simulink model "Model_5ms"  (Simulink 7.7)
settings: Solver=ode45  StartTime=0.0  StopTime=10.0  RelTol=1e-3
undefined symbols (not defined in the file): DiscIntNeverNeededParam
libraries: simulink x3, simulink_extras x2
settings Model: Creator=carsim  LastModifiedBy=jporter
settings DebuggingCC: FcnCallInpInsideContextMsg=Enable All

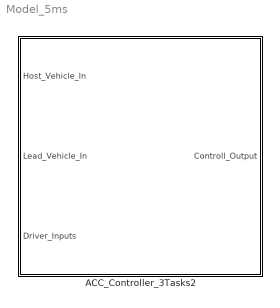
== system Model_5ms ==
  ACC_Controller_3Tasks2 : Subsystem

== system Model_5ms/ACC_Controller_3Tasks2 ==
  Host_Vehicle_In : Inport
  Lead_Vehicle_In : Inport  Port=2
  Driver_Inputs : Inport  Port=3
  HighLevelController : Subsystem
  Instrument Cluster : Subsystem
  LowLevel : Subsystem
  Mux2 : Mux  Inputs=5
  Controll_Output : Outport
  wires:
  Instrument Cluster/1(Detect) -> Mux2/3
  Instrument Cluster/2(Distance_actual) -> Mux2/4
  Mux2/1 -> Controll_Output/1
  Host_Vehicle_In/1 -> Instrument Cluster/1(Host_Vehicle_In)
  Driver_Inputs/1 -> Instrument Cluster/3(Driver_Inputs)
  Lead_Vehicle_In/1 -> Instrument Cluster/2(Lead_Vehicle_In)
  HighLevelController/1(To_LowLevelController) -> LowLevel/1(Lowlevel_inputs_from_HighLevel)
  Instrument Cluster/3(To_High_Level_Controller) -> HighLevelController/1(High_Level_inputs)
  LowLevel/1(Throttle_Angle) -> Instrument Cluster/4(Throttle_ang_in)
  LowLevel/2(P_mc_Brake) -> Instrument Cluster/5(P_mc_brake_in)
  LowLevel/3(desired_Range) -> Instrument Cluster/6(des_range_in)
  Instrument Cluster/4(Throttle_ang_out) -> Mux2/1
  Instrument Cluster/5(P_mc_brake_out) -> Mux2/2
  Instrument Cluster/6(des_range_out) -> Mux2/5

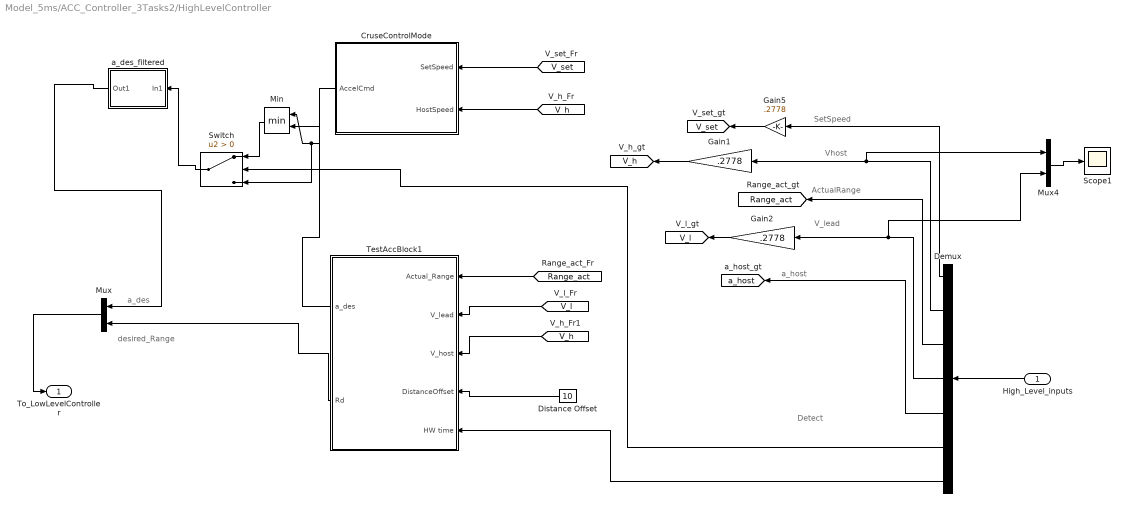
== system Model_5ms/ACC_Controller_3Tasks2/HighLevelController ==
  note: SetSpeed
  note: Vhost
  note: ActualRange
  note: V_lead
  note: a_host
  note: Detect
  note: a_des
  note: desired_Range
  High_Level_inputs : Inport
  CruseControlMode : Subsystem
  Demux : Demux  Outputs=7
  Distance Offset : Constant  Value=10
  Gain1 : Gain  Gain=.2778
  Gain2 : Gain  Gain=.2778
  Gain5 : Gain  Gain=.2778
  Min : MinMax  Inputs=2
  Mux : Mux  Inputs=2
  Mux4 : Mux  Inputs=2
  Scope1 : Scope
      settings: YMin=60  YMax=60.3
  Switch : Switch  Criteria=u2 > Threshold
  TestAccBlock1 : Subsystem
  a_des_filtered : Subsystem
  To_LowLevelController : Outport
  tag scope: Range_act=global, V_h=global, V_l=global, V_set=global, a_host=global
  wires:
  [V_h] -> TestAccBlock1/3(V_host)
  [V_h] -> CruseControlMode/2(HostSpeed)
  [V_set] -> CruseControlMode/1(SetSpeed)
  [Range_act] -> TestAccBlock1/1(Actual_Range)
  [V_l] -> TestAccBlock1/2(V_lead)
  Distance Offset/1 -> TestAccBlock1/4(DistanceOffset)
  CruseControlMode/1(AccelCmd) -> Switch/3, Min/1
  a_des_filtered/1(Out1) -> Mux/1
  TestAccBlock1/2(Rd) -> Mux/2
  TestAccBlock1/1(a_des) -> Min/2
  Switch/1 -> a_des_filtered/1(In1)
  Min/1 -> Switch/1
  Gain5/1 -> [V_set]
  Gain1/1 -> [V_h]
  Gain2/1 -> [V_l]
  Demux/7 -> TestAccBlock1/5(HW time)
  Demux/1 -> Gain5/1
  Demux/2 -> Gain1/1, Mux4/1
  Demux/3 -> [Range_act]
  Demux/4 -> Gain2/1, Mux4/2
  Demux/5 -> [a_host]
  Demux/6 -> Switch/2
  Mux/1 -> To_LowLevelController/1
  High_Level_inputs/1 -> Demux/1
  Mux4/1 -> Scope1/1

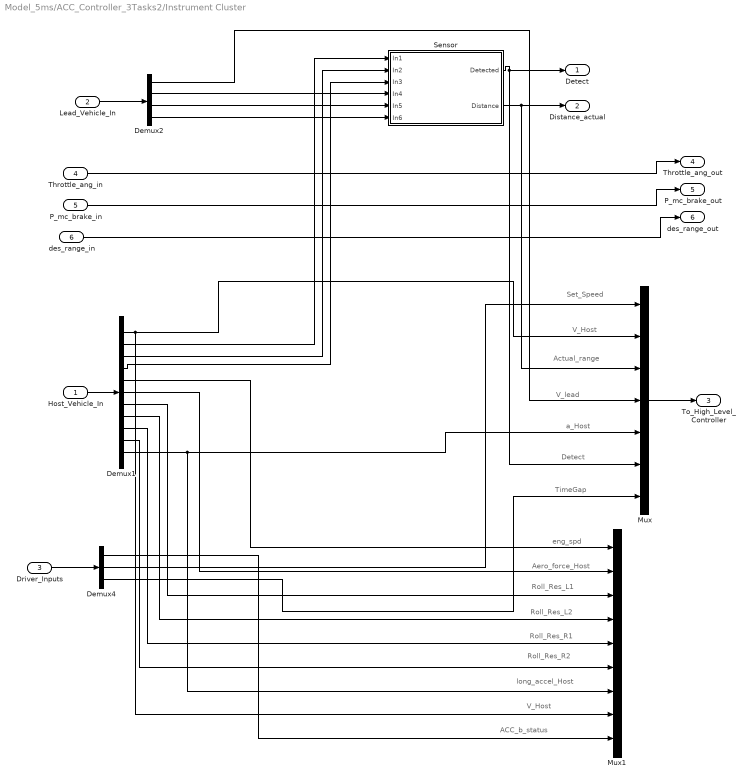
== system Model_5ms/ACC_Controller_3Tasks2/Instrument Cluster ==
  note: Set_Speed
  note: V_Host
  note: Actual_range
  note: V_lead
  note: a_Host
  note: Detect
  note: TimeGap
  note: eng_spd
  note: Aero_force_Host
  note: Roll_Res_L1
  note: Roll_Res_L2
  note: Roll_Res_R1
  note: Roll_Res_R2
  note: long_accel_Host
  note: V_Host
  note: ACC_b_status
  Host_Vehicle_In : Inport
  Lead_Vehicle_In : Inport  Port=2
  Driver_Inputs : Inport  Port=3
  Throttle_ang_in : Inport  Port=4
  P_mc_brake_in : Inport  Port=5
  des_range_in : Inport  Port=6
  Demux1 : Demux  Outputs=11
  Demux2 : Demux
  Demux4 : Demux  Outputs=3
  Mux : Mux  Inputs=7
  Mux1 : Mux  Inputs=9
  Sensor : Subsystem  mask{S_ANGLE=30, S_DISTANCE=100}
      mask prompts: S_ANGLE "View Angle (deg)"; S_DISTANCE "Distance Range (m)"
      mask help:
      | An example of a radar sensor. It can detect the distance between the sensor and another object according its position (Xo, Yo).
      |
      | Input parameters are View Angle(deg) and radar detectable distance(m).
      mask init:
      | d_ang= str2double(S_ANGLE)/2;
      | set_param([gcb '/View Angle'], 'Threshold', sprintf('%0.2f', d_ang));
      | set_param([gcb '/L-Radar'], 'Value', S_DISTANCE);
  Detect : Outport
  Distance_actual : Outport  Port=2
  To_High_Level_Controller : Outport  Port=3
  Throttle_ang_out : Outport  Port=4
  P_mc_brake_out : Outport  Port=5
  des_range_out : Outport  Port=6
  wires:
  Sensor/2(Distance) -> Distance_actual/1, Mux/3
  Sensor/1(Detected) -> Detect/1, Mux/6
  Demux4/1 -> Mux1/9
  Demux4/2 -> Mux/1
  Demux4/3 -> Mux/7
  Driver_Inputs/1 -> Demux4/1
  Demux1/1 -> Mux1/8, Mux/2
  Demux1/2 -> Sensor/1(In1)
  Demux1/3 -> Sensor/2(In2)
  Demux1/4 -> Sensor/3(In3)
  Demux1/5 -> Mux1/1
  Demux1/6 -> Mux1/2
  Demux1/7 -> Mux1/3
  Demux1/8 -> Mux1/4
  Demux1/9 -> Mux1/5
  Demux1/10 -> Mux1/6
  Demux1/11 -> Mux/5, Mux1/7
  Host_Vehicle_In/1 -> Demux1/1
  Lead_Vehicle_In/1 -> Demux2/1
  Demux2/2 -> Sensor/4(In4)
  Demux2/3 -> Sensor/5(In5)
  Demux2/4 -> Sensor/6(In6)
  Demux2/1 -> Mux/4
  Mux/1 -> To_High_Level_Controller/1
  Throttle_ang_in/1 -> Throttle_ang_out/1
  P_mc_brake_in/1 -> P_mc_brake_out/1
  des_range_in/1 -> des_range_out/1

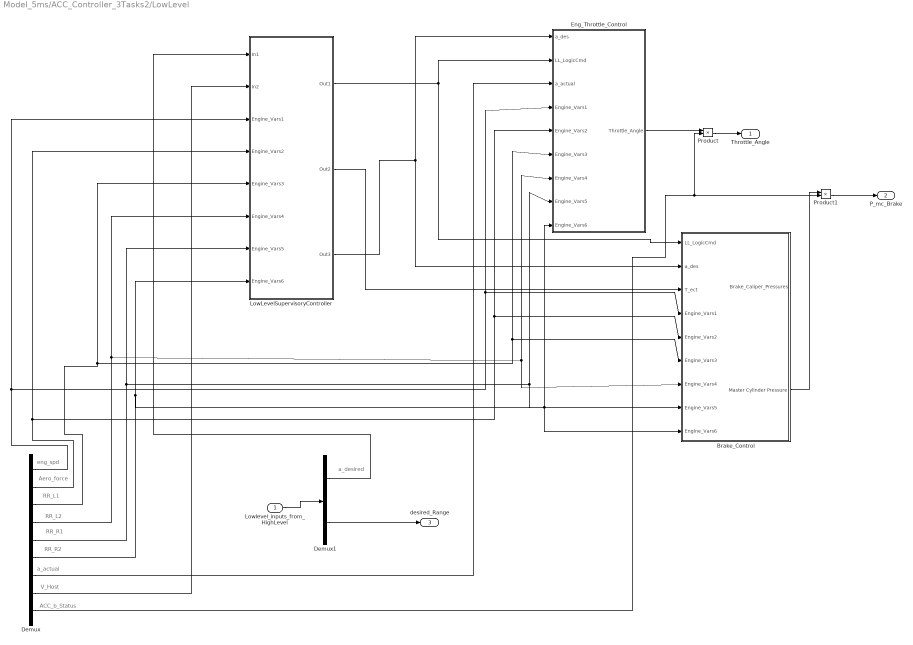
== system Model_5ms/ACC_Controller_3Tasks2/LowLevel ==
  note: eng_spd
  note: Aero_force
  note: RR_L1
  note: RR_L2
  note: RR_R1
  note: RR_R2
  note: a_desired
  note: a_actual
  note: V_Host
  note: ACC_b_Status
  Lowlevel_inputs_from_HighLevel : Inport
  Brake_Control : Subsystem
  Demux : Demux  Outputs=9
  Demux1 : Demux  Outputs=2
  Eng_Throttle_Control : Subsystem
  LowLevelSupervisoryController : Subsystem
  Product : Product  RndMeth=Zero
  Product1 : Product  RndMeth=Zero
  Throttle_Angle : Outport
  P_mc_Brake : Outport  Port=2
  desired_Range : Outport  Port=3
  wires:
  Demux/3 -> Eng_Throttle_Control/6(Engine_Vars3), Brake_Control/6(Engine_Vars3), LowLevelSupervisoryController/5(Engine_Vars3)
  Demux/5 -> Eng_Throttle_Control/8(Engine_Vars5), Brake_Control/8(Engine_Vars5), LowLevelSupervisoryController/7(Engine_Vars5)
  LowLevelSupervisoryController/1(Out1) -> Brake_Control/1(LL_LogicCmd), Eng_Throttle_Control/2(LL_LogicCmd)
  LowLevelSupervisoryController/3(Out3) -> Brake_Control/2(a_des), Eng_Throttle_Control/1(a_des)
  LowLevelSupervisoryController/2(Out2) -> Brake_Control/3(T_ect)
  Product/1 -> Throttle_Angle/1
  Product1/1 -> P_mc_Brake/1
  Eng_Throttle_Control/1(Throttle_Angle) -> Product/1
  Brake_Control/2(Master Cylinder Pressure) -> Product1/1
  Demux/1 -> Brake_Control/4(Engine_Vars1), Eng_Throttle_Control/4(Engine_Vars1), LowLevelSupervisoryController/3(Engine_Vars1)
  Demux/2 -> Eng_Throttle_Control/5(Engine_Vars2), Brake_Control/5(Engine_Vars2), LowLevelSupervisoryController/4(Engine_Vars2)
  Demux/4 -> Eng_Throttle_Control/7(Engine_Vars4), Brake_Control/7(Engine_Vars4), LowLevelSupervisoryController/6(Engine_Vars4)
  Demux/6 -> Eng_Throttle_Control/9(Engine_Vars6), Brake_Control/9(Engine_Vars6), LowLevelSupervisoryController/8(Engine_Vars6)
  Demux/9 -> Product/2, Product1/2
  Demux1/2 -> desired_Range/1
  Demux1/1 -> LowLevelSupervisoryController/1(In1)
  Demux/7 -> Eng_Throttle_Control/3(a_actual)
  Demux/8 -> LowLevelSupervisoryController/2(In2)
  Lowlevel_inputs_from_HighLevel/1 -> Demux1/1

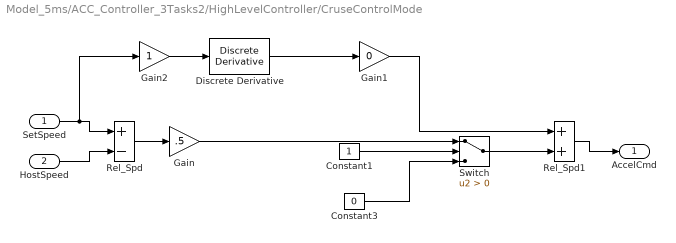
== system Model_5ms/ACC_Controller_3Tasks2/HighLevelController/CruseControlMode ==
  SetSpeed : Inport
  HostSpeed : Inport  Port=2
  Constant1 : Constant
  Constant3 : Constant  Value=0
  Discrete Derivative : simulink/Discrete/Discrete Derivative  gainval=.1  ICPrevScaledInput=0.0  InputProcessing=Inherited  OutMin=[]  OutMax=[]  OutDataType=fixdt(1, 16)  OutScaling=2^-10  DoSatur=off
  Gain : Gain  Gain=.5
  Gain1 : Gain  Gain=0
  Gain2 : Gain  SampleTime=.005
  Rel_Spd : Sum  Inputs=+-
  Rel_Spd1 : Sum
  Switch : Switch  Criteria=u2 > Threshold
  AccelCmd : Outport
  wires:
  SetSpeed/1 -> Rel_Spd/1, Gain2/1
  HostSpeed/1 -> Rel_Spd/2
  Rel_Spd/1 -> Gain/1
  Gain/1 -> Switch/1
  Constant3/1 -> Switch/3
  Switch/1 -> Rel_Spd1/2
  Constant1/1 -> Switch/2
  Gain1/1 -> Rel_Spd1/1
  Discrete Derivative/1 -> Gain1/1
  Rel_Spd1/1 -> AccelCmd/1
  Gain2/1 -> Discrete Derivative/1

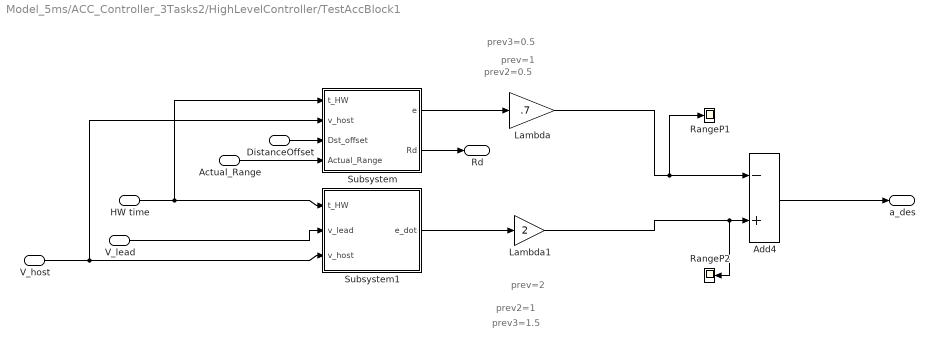
== system Model_5ms/ACC_Controller_3Tasks2/HighLevelController/TestAccBlock1 ==
  note: prev=1
  note: prev=2
  note: prev2=0.5
  note: prev2=1
  note: prev3=1.5
  note: prev3=0.5
  Actual_Range : Inport
  V_lead : Inport  Port=2
  V_host : Inport  Port=3
  DistanceOffset : Inport  Port=4
  HW time : Inport  Port=5
  Add4 : Sum  Inputs=-+
  Lambda : Gain  Gain=.7
  Lambda1 : Gain  Gain=2
  RangeP1 : Scope
      settings: TickLabels=on  TimeRange=50  YMin=-2  YMax=3.75  SaveName=ScopeData32  DataFormat=Array  SampleTime=100
  RangeP2 : Scope
      settings: TickLabels=on  TimeRange=50  YMin=-2  YMax=3.75  SaveName=ScopeData33  DataFormat=Array  SampleTime=100
  Subsystem : Subsystem
  Subsystem1 : Subsystem
  a_des : Outport
  Rd : Outport  Port=2
  wires:
  V_host/1 -> Subsystem1/3(v_host), Subsystem/2(v_host)
  HW time/1 -> Subsystem1/1(t_HW), Subsystem/1(t_HW)
  V_lead/1 -> Subsystem1/2(v_lead)
  Subsystem1/1(e_dot) -> Lambda1/1
  Lambda/1 -> Add4/1, RangeP1/1
  Add4/1 -> a_des/1
  Subsystem/1(e) -> Lambda/1
  Actual_Range/1 -> Subsystem/4(Actual_Range)
  DistanceOffset/1 -> Subsystem/3(Dst_offset)
  Subsystem/2(Rd) -> Rd/1
  Lambda1/1 -> Add4/2, RangeP2/1

== system Model_5ms/ACC_Controller_3Tasks2/HighLevelController/a_des_filtered ==
  In1 : Inport
  Discrete Transfer Fcn : DiscreteTransferFcn  Numerator=[0,0.00120910427425029,0.00116946476028127]  Denominator=[1,-1.90245884900143,0.904837418035960]  SampleTime=.005
  Saturation : Saturate  UpperLimit=2  LowerLimit=-3
  Out1 : Outport
  wires:
  In1/1 -> Saturation/1
  Discrete Transfer Fcn/1 -> Out1/1
  Saturation/1 -> Discrete Transfer Fcn/1

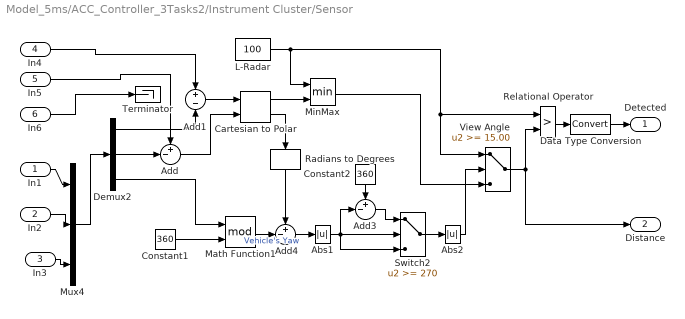
== system Model_5ms/ACC_Controller_3Tasks2/Instrument Cluster/Sensor ==
  In1 : Inport
  In2 : Inport  Port=2
  In3 : Inport  Port=3
  In4 : Inport  Port=4
  In5 : Inport  Port=5
  In6 : Inport  Port=6
  Abs1 : Abs
  Abs2 : Abs
  Add : Sum  Inputs=+-|
  Add1 : Sum  Inputs=+-
  Add3 : Sum  Inputs=+-|
  Add4 : Sum  Inputs=+-|
  Cartesian to Polar : simulink_extras/Transformations/Cartesian to Polar
  Constant1 : Constant  Value=360
  Constant2 : Constant  Value=360
  Data Type Conversion : DataTypeConversion  RndMeth=Zero
  Demux2 : Demux  Outputs=3
  L-Radar : Constant  Value=100
  Math Function1 : Math  Operator=mod  SaturateOnIntegerOverflow=on
  MinMax : MinMax  Inputs=2  SaturateOnIntegerOverflow=on  InputSameDT=on
  Mux4 : Mux  Inputs=3
  Radians to Degrees : simulink_extras/Transformations/Radians to Degrees
  Relational Operator : RelationalOperator  Operator=>  OutDataTypeStr=boolean
  Switch2 : Switch  Threshold=270
  Terminator : Terminator
  View Angle : Switch  Threshold=15.00
  Detected : Outport
  Distance : Outport  Port=2
  wires:
  Demux2/3 -> Math Function1/1
  Constant1/1 -> Math Function1/2
  Add/1 -> Cartesian to Polar/2
  Add1/1 -> Cartesian to Polar/1
  Demux2/1 -> Add1/2
  In4/1 -> Add1/1
  Demux2/2 -> Add/2
  In5/1 -> Add/1
  In6/1 -> Terminator/1
  Math Function1/1 -> Add4/2  "Vehicle's Yaw"
  Add4/1 -> Abs1/1
  Abs1/1 -> Switch2/2, Add3/2, Switch2/3
  Add3/1 -> Switch2/1
  Constant2/1 -> Add3/1
  L-Radar/1 -> MinMax/1, View Angle/1, Relational Operator/1
  MinMax/1 -> View Angle/3
  Switch2/1 -> Abs2/1
  Abs2/1 -> View Angle/2
  View Angle/1 -> Distance/1, Relational Operator/2
  Relational Operator/1 -> Data Type Conversion/1
  Data Type Conversion/1 -> Detected/1
  Radians to Degrees/1 -> Add4/1
  Cartesian to Polar/1 -> MinMax/2
  Cartesian to Polar/2 -> Radians to Degrees/1
  Mux4/1 -> Demux2/1
  In1/1 -> Mux4/1
  In2/1 -> Mux4/2
  In3/1 -> Mux4/3

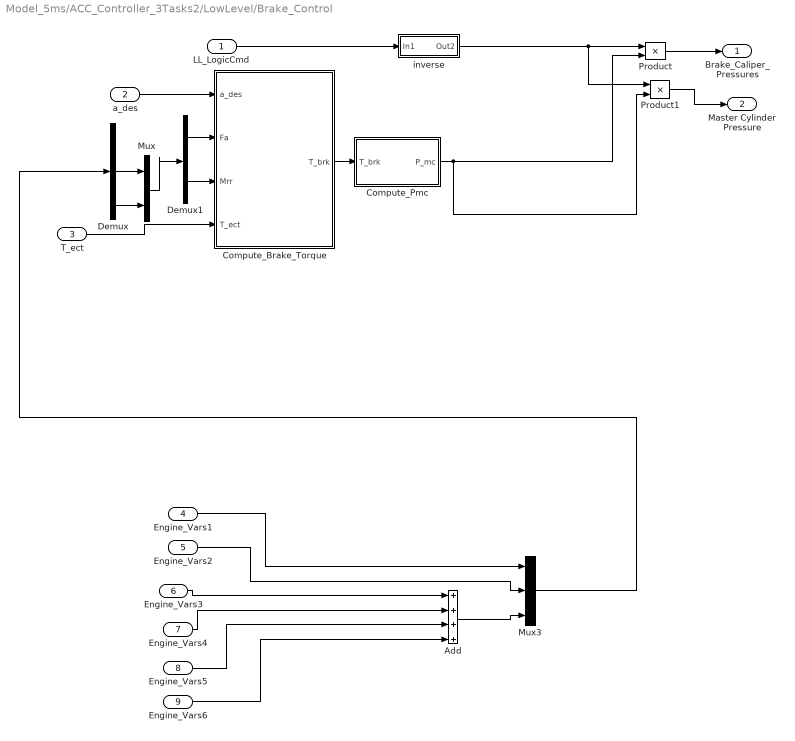
== system Model_5ms/ACC_Controller_3Tasks2/LowLevel/Brake_Control ==
  LL_LogicCmd : Inport
  a_des : Inport  Port=2
  T_ect : Inport  Port=3
  Engine_Vars1 : Inport  Port=4
  Engine_Vars2 : Inport  Port=5
  Engine_Vars3 : Inport  Port=6
  Engine_Vars4 : Inport  Port=7
  Engine_Vars5 : Inport  Port=8
  Engine_Vars6 : Inport  Port=9
  Add : Sum  Inputs=++++
  Compute_Brake_Torque : Stateflow chart  TreatAsAtomicUnit=on
  Compute_Pmc : Stateflow chart  TreatAsAtomicUnit=on
  Demux : Demux  Outputs=3
  Demux1 : Demux  Outputs=2
  Mux : Mux  Inputs=2
  Mux3 : Mux  Inputs=3
  Product : Product  RndMeth=Zero
  Product1 : Product  RndMeth=Zero
  inverse : Subsystem
  Brake_Caliper_Pressures : Outport
  Master Cylinder Pressure : Outport  Port=2
  wires:
  LL_LogicCmd/1 -> inverse/1(In1)
  inverse/1(Out2) -> Product/1, Product1/1
  Product/1 -> Brake_Caliper_Pressures/1
  Mux3/1 -> Demux/1
  Compute_Pmc/1(P_mc) -> Product1/2, Product/2
  Product1/1 -> Master Cylinder Pressure/1
  Compute_Brake_Torque/1(T_brk) -> Compute_Pmc/1(T_brk)
  Demux1/1 -> Compute_Brake_Torque/2(Fa)
  Demux1/2 -> Compute_Brake_Torque/3(Mrr)
  Demux/3 -> Mux/2
  Demux/2 -> Mux/1
  Mux/1 -> Demux1/1
  T_ect/1 -> Compute_Brake_Torque/4(T_ect)
  a_des/1 -> Compute_Brake_Torque/1(a_des)
  Engine_Vars2/1 -> Mux3/2
  Engine_Vars3/1 -> Add/1
  Engine_Vars4/1 -> Add/2
  Add/1 -> Mux3/3
  Engine_Vars1/1 -> Mux3/1
  Engine_Vars5/1 -> Add/3
  Engine_Vars6/1 -> Add/4

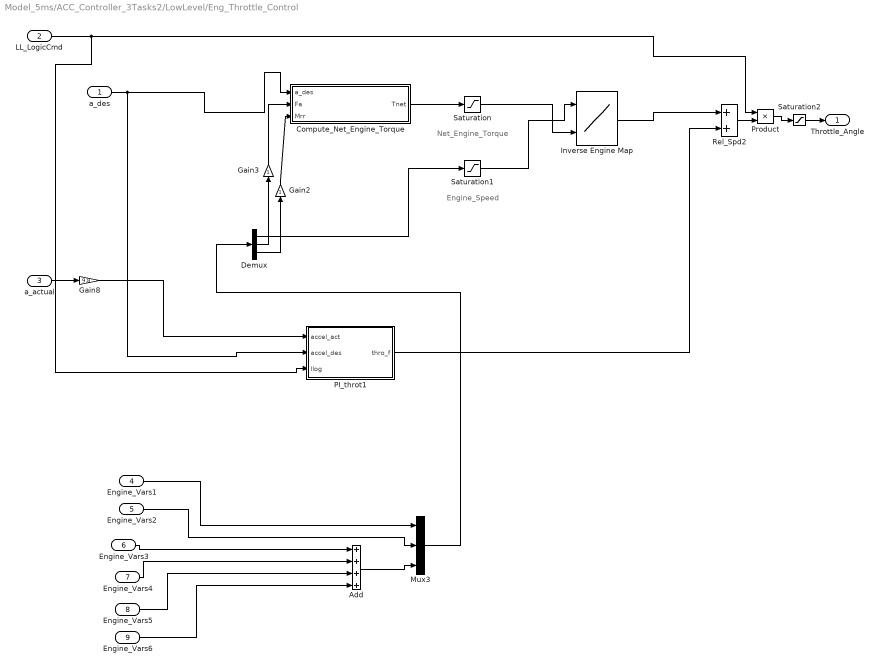
== system Model_5ms/ACC_Controller_3Tasks2/LowLevel/Eng_Throttle_Control ==
  note: Net_Engine_Torque
  note: Engine_Speed
  a_des : Inport
  LL_LogicCmd : Inport  Port=2
  a_actual : Inport  Port=3
  Engine_Vars1 : Inport  Port=4
  Engine_Vars2 : Inport  Port=5
  Engine_Vars3 : Inport  Port=6
  Engine_Vars4 : Inport  Port=7
  Engine_Vars5 : Inport  Port=8
  Engine_Vars6 : Inport  Port=9
  Add : Sum  Inputs=++++
  Compute_Net_Engine_Torque : Stateflow chart  TreatAsAtomicUnit=on
  Demux : Demux  Outputs=3
  Gain2 : Gain
  Gain3 : Gain
  Gain8 : Gain  Gain=9.8
  Inverse Engine Map : Lookup_n-D  BreakpointsForDimension1=|  BreakpointsForDimension2=[-131:12:514]  Table=[0,0,0,0,0,0,0,0,0,0,0,0,0,0,0,0.0100000000000000,0.0200000000000000,0.0400000000000000,0.0500000000000000,0.0700000000000000,0.0800000000000000,0.0900000000000000,0.110000000000000,0.120000000000000,0.140000000000000,0.160000000000000,0.950000000000000,0.950000000000000,0.950000000000000,0.950000000000000,0.950000000000000,0.950000000000000,0.950000000000000,0.950000000000000,0.950000000000000,0.950000000000000,0.950000000000000,0.950000000000000,0.950000000000000,0.950000000000000,0.950000000000000,0.950000000000000,0.950000000000000,0.950000000000000,0.950000000000000,0.950000000000000,0.950000000000000,0.950000000000000,0.950000000000000,0.950000000000000,0.950000000000000,0.950000000000000,0.950000000000000,0.950000000000000;0,0,0,0,0,0,0,0,0,0,0,0,0,0,0,0,0.0100000000000000,0.0200000000000000,0.0300000000000000,0.0500000000000000,0.0600000000000000,0.0700000000000000,0.0800000000000000,0.0900000000000000,0.100000000000000,0.110000000000000,0.120000000000000,0.120000000000000,0.130000000000000,0.140000000000000,0.150000000000000,0.180000000000000,1,1,1,1,1,1,1,1,1,1,1,1,1,1,1,1,1,1,1,1,1,1;0,0,0,0,0,0,0,0,0,0,0,0,0.0100000000000000,0.0200000000000000,0.0300000000000000,0.0300000000000000,0.0400000000000000,0.0500000000000000,0.0600000000000000,0.0700000000000000,0.0800000000000000,0.0800000000000000,0.0900000000000000,0.100000000000000,0.110000000000000,0.110000000000000,0.120000000000000,0.120000000000000,0.130000000000000,0.140000000000000,0.140000000000000,0.150000000000000,0.170000000000000,0.190000000000000,0.690000000000000,0.850000000000000,0.850000000000000,0.850000000000000,0.850000000000000,0.850000000000000,0.850000000000000,0.850000000000000,0.850000000000000,0.850000000000000,0.850000000000000,0.850000000000000,0.850000000000000,0.850000000000000,0.850000000000000,0.850000000000000,0.850000000000000,0.850000000000000,0.850000000000000,0.850000000000000;0,0,0,0,0,0,0,0,0,0,0,0.0100000000000000,0.0200000000000000,0.0300000000000000,0.0400000000000000,0.0500000000000000,0.0600000000000000,0.0700000000000000,0.0800000000000000,0.0800000000000000,0.0900000000000000,0.100000000000000,0.100000000000000,0.110000000000000,0.110000000000000,0.120000000000000,0.120000000000000,0.120000000000000,0.130000000000000,0.130000000000000,0.130000000000000,0.140000000000000,0.140000000000000,0.140000000000000,0.150000000000000,0.150000000000000,0.170000000000000,0.180000000000000,0.190000000000000,0.260000000000000,0.410000000000000,0.850000000000000,0.850000000000000,0.850000000000000,0.850000000000000,0.850000000000000,0.850000000000000,0.850000000000000,0.850000000000000,0.850000000000000,0.850000000000000,0.850000000000000,0.850000000000000,0.850000000000000;0,0,0,0,0,0,0,0,0,0,0.0100000000000000,0.0200000000000000,0.0400000000000000,0.0500000000000000,0.0600000000000000,0.0700000000000000,0.0800000000000000,0.0900000000000000,0.100000000000000,0.100000000000000,0.110000000000000,0.110000000000000,0.110000000000000,0.120000000000000,0.120000000000000,0.120000000000000,0.130000000000000,0.130000000000000,0.130000000000000,0.130000000000000,0.140000000000000,0.140000000000000,0.140000000000000,0.150000000000000,0.150000000000000,0.160000000000000,0.170000000000000,0.180000000000000,0.180000000000000,0.190000000000000,0.220000000000000,0.310000000000000,0.430000000000000,0.960000000000000,1,1,1,1,1,1,1,1,1,1;0,0,0,0,0,0,0,0,0,0.0100000000000000,0.0200000000000000,0.0400000000000000,0.0600000000000000,0.0700000000000000,0.0900000000000000,0.100000000000000,0.100000000000000,0.110000000000000,0.110000000000000,0.110000000000000,0.120000000000000,0.120000000000000,0.120000000000000,0.130000000000000,0.130000000000000,0.130000000000000,0.130000000000000,0.140000000000000,0.140000000000000,0.140000000000000,0.150000000000000,0.150000000000000,0.150000000000000,0.160000000000000,0.160000000000000,0.170000000000000,0.180000000000000,0.180000000000000,0.190000000000000,0.190000000000000,0.200000000000000,0.240000000000000 ...(+10120 chars)]  RndMeth=Simplest  InputSameDT=on
      | [517
      | 633
      | 750
      | 1107
      | 1463
      | 1820
      | 2177
      | 2533
      | 2890
      | 3247
      | 3603
      | 3960
      | 4317
      | 4673
      | 5030
      | 5387
      | 5743
      | 6100]
  Mux3 : Mux  Inputs=3
  PI_throt1 : Subsystem
  Product : Product  RndMeth=Zero
  Rel_Spd2 : Sum
  Saturation : Saturate  UpperLimit=514  LowerLimit=-131
  Saturation1 : Saturate  UpperLimit=6100  LowerLimit=0
  Saturation2 : Saturate  UpperLimit=1  LowerLimit=0
  Throttle_Angle : Outport
  wires:
  LL_LogicCmd/1 -> PI_throt1/3(llog), Product/1
  Inverse Engine Map/1 -> Rel_Spd2/1
  Demux/1 -> Saturation1/1
  Compute_Net_Engine_Torque/1(Tnet) -> Saturation/1
  a_des/1 -> Compute_Net_Engine_Torque/1(a_des), PI_throt1/2(accel_des)
  Demux/2 -> Gain3/1
  Demux/3 -> Gain2/1
  Gain2/1 -> Compute_Net_Engine_Torque/3(Mrr)
  Gain3/1 -> Compute_Net_Engine_Torque/2(Fa)
  Saturation/1 -> Inverse Engine Map/2
  Saturation1/1 -> Inverse Engine Map/1
  PI_throt1/1(thro_f) -> Rel_Spd2/2
  Rel_Spd2/1 -> Product/2
  Saturation2/1 -> Throttle_Angle/1
  Product/1 -> Saturation2/1
  a_actual/1 -> Gain8/1
  Gain8/1 -> PI_throt1/1(accel_act)
  Engine_Vars2/1 -> Mux3/2
  Engine_Vars3/1 -> Add/1
  Engine_Vars4/1 -> Add/2
  Add/1 -> Mux3/3
  Engine_Vars1/1 -> Mux3/1
  Engine_Vars5/1 -> Add/3
  Engine_Vars6/1 -> Add/4
  Mux3/1 -> Demux/1

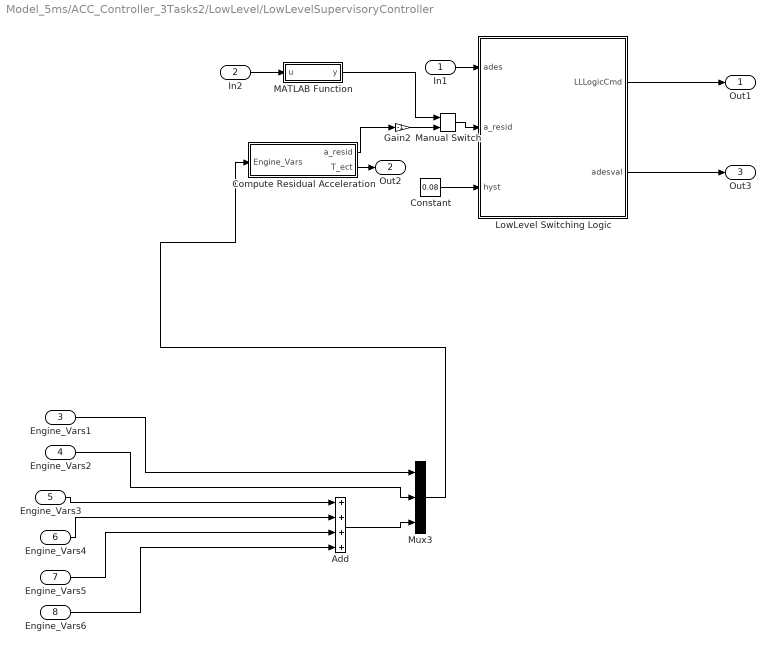
== system Model_5ms/ACC_Controller_3Tasks2/LowLevel/LowLevelSupervisoryController ==
  In1 : Inport
  In2 : Inport  Port=2
  Engine_Vars1 : Inport  Port=3
  Engine_Vars2 : Inport  Port=4
  Engine_Vars3 : Inport  Port=5
  Engine_Vars4 : Inport  Port=6
  Engine_Vars5 : Inport  Port=7
  Engine_Vars6 : Inport  Port=8
  Add : Sum  Inputs=++++
  Compute Residual Acceleration : Subsystem
  Constant : Constant  Value=0.08
  Gain2 : Gain  Gain=-1
  LowLevel Switching Logic : Stateflow chart  TreatAsAtomicUnit=on
  MATLAB Function : Stateflow chart  TreatAsAtomicUnit=on
  Manual Switch : simulink/Signal Routing/Manual Switch  sw=1  action=0  varsize=off
  Mux3 : Mux  Inputs=3
  Out1 : Outport
  Out2 : Outport  Port=2
  Out3 : Outport  Port=3
  wires:
  Compute Residual Acceleration/1(a_resid) -> Gain2/1
  Constant/1 -> LowLevel Switching Logic/3(hyst)
  Manual Switch/1 -> LowLevel Switching Logic/2(a_resid)
  Gain2/1 -> Manual Switch/2
  MATLAB Function/1(y) -> Manual Switch/1
  In2/1 -> MATLAB Function/1(u)
  In1/1 -> LowLevel Switching Logic/1(ades)
  LowLevel Switching Logic/1(LLLogicCmd) -> Out1/1
  Compute Residual Acceleration/2(T_ect) -> Out2/1
  LowLevel Switching Logic/2(adesval) -> Out3/1
  Engine_Vars2/1 -> Mux3/2
  Engine_Vars3/1 -> Add/1
  Engine_Vars4/1 -> Add/2
  Add/1 -> Mux3/3
  Engine_Vars1/1 -> Mux3/1
  Engine_Vars5/1 -> Add/3
  Engine_Vars6/1 -> Add/4
  Mux3/1 -> Compute Residual Acceleration/1(Engine_Vars)

== system Model_5ms/ACC_Controller_3Tasks2/HighLevelController/TestAccBlock1/Subsystem ==
  t_HW : Inport
  v_host : Inport  Port=2
  Dst_offset : Inport  Port=3
  Actual_Range : Inport  Port=4
  CmpDesRange : Sum  Inputs=+-
  DEsired Range : Subsystem
  e : Outport
  Rd : Outport  Port=2
  wires:
  v_host/1 -> DEsired Range/2(v_host)
  t_HW/1 -> DEsired Range/1(t_HW)
  Dst_offset/1 -> DEsired Range/3(Dst_offset)
  Actual_Range/1 -> CmpDesRange/2
  CmpDesRange/1 -> e/1
  DEsired Range/1(R_d) -> CmpDesRange/1, Rd/1

== system Model_5ms/ACC_Controller_3Tasks2/HighLevelController/TestAccBlock1/Subsystem1 ==
  t_HW : Inport
  v_lead : Inport  Port=2
  v_host : Inport  Port=3
  CmpDesRange1 : Sum  Inputs=+-
  e_dot : Outport
  wires:
  v_lead/1 -> CmpDesRange1/1
  v_host/1 -> CmpDesRange1/2
  CmpDesRange1/1 -> e_dot/1

== system Model_5ms/ACC_Controller_3Tasks2/LowLevel/Brake_Control/inverse ==
  In1 : Inport
  add : Sum  Inputs=+-
  cnst : Constant
  Out2 : Outport
  wires:
  cnst/1 -> add/1
  add/1 -> Out2/1
  In1/1 -> add/2

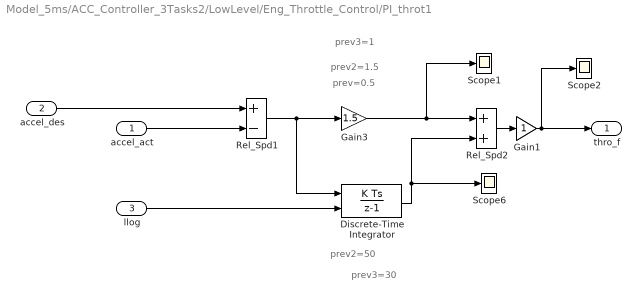
== system Model_5ms/ACC_Controller_3Tasks2/LowLevel/Eng_Throttle_Control/PI_throt1 ==
  note: prev=0.5
  note: prev2=50
  note: prev2=1.5
  note: prev3=30
  note: prev3=1
  accel_act : Inport
  accel_des : Inport  Port=2
  llog : Inport  Port=3
  Discrete-Time Integrator : DiscreteIntegrator  gainval=40  ExternalReset=either  SampleTime=.005  ICPrevOutput=DiscIntNeverNeededParam  ICPrevScaledInput=DiscIntNeverNeededParam
  Gain1 : Gain
  Gain3 : Gain  Gain=1.5
  Rel_Spd1 : Sum  Inputs=+-
  Rel_Spd2 : Sum
  Scope1 : Scope
      settings: YMin=0.0809  YMax=0.08155  SaveName=ScopeData36
  Scope2 : Scope
      settings: YMin=-2.8  YMax=-1.7  SaveName=ScopeData37
  Scope6 : Scope
      settings: YMin=0.217  YMax=0.22075  SaveName=ScopeData35
  thro_f : Outport
  wires:
  accel_des/1 -> Rel_Spd1/1
  accel_act/1 -> Rel_Spd1/2
  Rel_Spd1/1 -> Gain3/1, Discrete-Time Integrator/1
  Gain3/1 -> Rel_Spd2/1, Scope1/1
  Rel_Spd2/1 -> Gain1/1
  Discrete-Time Integrator/1 -> Rel_Spd2/2, Scope6/1
  llog/1 -> Discrete-Time Integrator/2
  Gain1/1 -> thro_f/1, Scope2/1

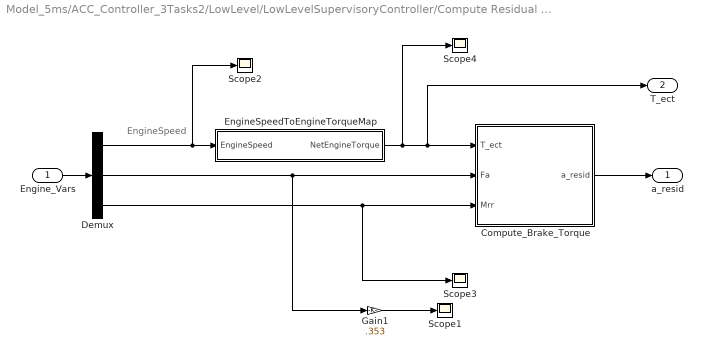
== system Model_5ms/ACC_Controller_3Tasks2/LowLevel/LowLevelSupervisoryController/Compute Residual Acceleration ==
  note: EngineSpeed
  Engine_Vars : Inport
  Compute_Brake_Torque : Stateflow chart  TreatAsAtomicUnit=on
  Demux : Demux  Outputs=3
  EngineSpeedToEngineTorqueMap : Subsystem
  Gain1 : Gain  Gain=.353
  Scope{1..4} (4 alike) : Scope
      Scope1 settings: YMin=-12.7  YMax=-11.6  SaveName=ScopeData44
      Scope2 settings: YMin=0.177  YMax=0.1795  SaveName=ScopeData45
      Scope3 settings: YMin=-27.5607  YMax=-27.5577  SaveName=ScopeData43
      Scope4 settings: YMin=2.82755  YMax=2.8276  SaveName=ScopeData46
  a_resid : Outport
  T_ect : Outport  Port=2
  wires:
  Engine_Vars/1 -> Demux/1
  Demux/2 -> Compute_Brake_Torque/2(Fa), Gain1/1
  Demux/3 -> Compute_Brake_Torque/3(Mrr), Scope3/1
  Compute_Brake_Torque/1(a_resid) -> a_resid/1
  EngineSpeedToEngineTorqueMap/1(NetEngineTorque) -> Compute_Brake_Torque/1(T_ect), T_ect/1, Scope4/1
  Demux/1 -> EngineSpeedToEngineTorqueMap/1(EngineSpeed), Scope2/1
  Gain1/1 -> Scope1/1

== system Model_5ms/ACC_Controller_3Tasks2/HighLevelController/TestAccBlock1/Subsystem/DEsired Range ==
  t_HW : Inport
  v_host : Inport  Port=2
  Dst_offset : Inport  Port=3
  CmpDesRange : Sum
  Product : Product  RndMeth=Zero
  R_d : Outport
  wires:
  t_HW/1 -> Product/1
  v_host/1 -> Product/2
  Product/1 -> CmpDesRange/1
  Dst_offset/1 -> CmpDesRange/2
  CmpDesRange/1 -> R_d/1

== system Model_5ms/ACC_Controller_3Tasks2/LowLevel/LowLevelSupervisoryController/Compute Residual Acceleration/EngineSpeedToEngineTorqueMap ==
  EngineSpeed : Inport
  EngineMap1 : simulink/Lookup Tables/Lookup Table Dynamic  LookUpMeth=Interpolation-Use End Values  OutDataTypeStr=fixdt('double')  OutputDataTypeScalingMode=Specify via dialog  OutDataType=fixdt('double')  OutScaling=2^-10  DoSatur=off
  EngineSpeedTable1 : Constant  Value=|
      | [0
      | 400
      | 517
      | 633
      | 750
      | 1107
      | 1463
      | 1820
      | 2177
      | 2533
      | 2890
      | 3247
      | 3603
      | 3960
      | 4317
      | 4673
      | 5030
      | 5387
      | 5743
      | 6100
      | 6500
      | 6700]
  NetEngineTorqueTable1 : Constant  Value=|
      | [0
      | 0
      | 41.1300
      | 49.3500
      | 0
      | -16.4500
      | -24.6800
      | -27.9700
      | -33.5100
      | -42.0700
      | -50.0800
      | -57.1400
      | -64.0800
      | -71.0600
      | -78.4400
      | -86.1100
      | -94.2800
      | -102.4700
      | -111.6500
      | -121.6500
      | -133.2500
      | -134.8900]
  NetEngineTorque : Outport
  wires:
  EngineSpeedTable1/1 -> EngineMap1/2
  NetEngineTorqueTable1/1 -> EngineMap1/3
  EngineSpeed/1 -> EngineMap1/1
  EngineMap1/1 -> NetEngineTorque/1

== matlab function ACC_Controller_3Tasks2/LowLevel/Brake_Control/Compute_Brake_Torque ==
  data: a_des input double; T_brk output double; Fa input double; Mrr input double; T_ect input double
function T_brk = fcn(a_des,Fa,Mrr,T_ect)
%#codegen
%Source: Coordinated Adaptive Cruise Control: Design and Simulation by Michael Christopher Drew
Beta=582.74;%928.1; %Beta is the lumped Inertia
Rg=1.37*(2.65);%4;%Rg is Gear Ratio
%Mrr=0;%Mrr is the Rolling Resistance Torque
h=.3530;%h is Effective Wheel Radius
%Fa=0;%Fa is Aerodynamic Drag Force
m=1650; %m is the lumped mass of the vehicle
g=9.8; %g is acceleration due to gravity
theta=0; %theta is the road grade or incline
%T_brk= (Beta*a_des)+(Rg*(Mrr+(h*Fa)+(m*g*h*sin(theta))));
%T_brk= -((1/Rg)*((Beta*a_des)+T_ect))-(Mrr+(h*Fa)+(m*g*sin(theta)));
T_brk= -((1/Rg)*((Beta*a_des)+T_ect))+(Mrr+(h*Fa)+(m*g*sin(theta)));

== matlab function ACC_Controller_3Tasks2/LowLevel/Brake_Control/Compute_Pmc ==
  data: T_brk input double; P_mc output double
function P_mc = fcn(T_brk)
%#codegen
%Relationship between T_brk and Pmc
%T_brk=Kb(Pmc-Ppo)
%where
%Pmc is the master cylinder pressure
Kb=800;%50;%200;%350;%Kb is the brake gain
Ppo=0;%Ppo is the push-out pressure require to engage brake

P_mc=(T_brk/Kb)+Ppo;

== matlab function ACC_Controller_3Tasks2/LowLevel/Eng_Throttle_Control/Compute_Net_Engine_Torque ==
  data: a_des input double; Tnet output double; Fa input double; Mrr input double
function Tnet = fcn(a_des,Fa,Mrr)
%#codegen
Beta=582.71;%928.1; %Beta is the lumped Inertia
Rg=1.37*(2.65);%4;%Rg is Gear Ratio
%Mrr=0;%Mrr is the Rolling Resistance Torque
h=.3530;%h is Effective Wheel Radius
%Fa=0;%Fa is Aerodynamic Drag Force
m=1650; %m is the lumped mass of the vehicle
g=9.8; %g is acceleration due to gravity
theta=0; %theta is the road grade or incline
%Tnet= (Beta*a_des)+(Rg*(Mrr+(h*Fa)+(m*g*h*sin(theta))));
Tnet= (Beta*a_des)-(Rg*(Mrr+(h*Fa)+(m*g*h*sin(theta))));
%Tnet= (Rg*m*a_des)+(Rg*(Mrr+(h*Fa)+(m*g*h*sin(theta))));

== matlab function ACC_Controller_3Tasks2/LowLevel/LowLevelSupervisoryController/Compute Residual Acceleration/Compute_Brake_Torque ==
  data: T_ect input double; a_resid output double; Fa input double; Mrr input double
function a_resid = fcn(T_ect,Fa,Mrr)
%#codegen
Beta=582.74;%928.1; %Beta is the lumped Inertia
Rg=1.37*(2.65);%4;%Rg is Gear Ratio
%Mrr is the Rolling Resistance Torque
h=.3530;%h is Effective Wheel Radius
%Fa is Aerodynamic Drag Force
m=1650; %m is the lumped mass of the vehicle
g=9.8; %g is acceleration due to gravity
theta=0; %theta is the road grade or incline
a_resid=(1/Beta)*(T_ect+(Rg*(Mrr+(h*Fa)+(m*g*sin(theta)))));

== stateflow chart ACC_Controller_3Tasks2/LowLevel/LowLevelSupervisoryController/LowLevel Switching Logic ==
  state EngThrottleControl
    during:adesval=ades;LLLogicCmd=1;
  state BrakeControl
    during:adesval=ades;;LLLogicCmd=0;
  (default) -> EngThrottleControl
  BrakeControl -> EngThrottleControl : [ades>=(a_resid+hyst)]/adesval=ades;LLLogicCmd=1
  EngThrottleControl -> BrakeControl : [ades<(a_resid-hyst)]/adesval=ades;LLLogicCmd=0
  data: LLLogicCmd output double; ades input double; adesval output double; a_resid input double; hyst input double

== matlab function ACC_Controller_3Tasks2/LowLevel/LowLevelSupervisoryController/MATLAB Function ==
  data: u input double; y output double
function y = fcn(u)
%#codegen
Vrel=[120 110 100 90 80 70 60 50 40 30 20 10];
Accelre=[-1.64 -1.4 -1.2 -1.01 -0.83 -0.7 -.57 -0.47 -0.37 -0.3 -.23 -0.186];

y=interp1(Vrel,Accelre,u);
